simulink library "legs"  (R2020b)
settings: Solver=VariableStepAuto  StartTime=0.0  StopTime=10.0  RelTol=1e-3
values from neighbouring files (symbols this model uses):
  N = size(waypoints, 1)    [interpolate_leg_waypoints.m]
undefined symbols (not defined in the file or in its folder): beta, X, Y, Z
libraries: sm_lib x42, $bdroot x21, nesl_utility x9
(part 2 of 2)

== stateflow chart legs/Quadruped Walk Gait/Leg 2 Gait ==
  state Initial_
    entry:
    u_start = u;
    u_elapsed = 0;
    during:
    u_elapsed = u - u_start;
  state Lifted
    entry:
    N = 10;
    waypoints = leg_waypoints(config, contact_start_config, N);
    u_start = u;
    u_elapsed = 0;
    velocity_control = 0;
    during:
    i = ceil((u_elapsed/(1-beta))*N);
    config_cmd = waypoints(i);
  state Contact
    entry:
    u_start = u;
    u_elapsed = 0;
    velocity_control = 1;
    during:
    config_dot_cmd = leg_config_dot_ik(config, vx, vy, omega);
    u_elapsed = u - u_start;
  (default) -> Initial_
  Initial_ -> Contact : [u_elapsed > phi]
  Contact -> Lifted : [u_elapsed > beta]
  Lifted -> Contact : [u_elapsed > (1-beta)]
  data: config_cmd output; config_dot_cmd output; vx input; vy input; omega input; u input; velocity_control output; N local; config input; i local; u_elapsed local; u_start local; waypoints local; contact_start_config input; phi input; beta input
